simulink model "Alternative_VTOLAutopilotController"  (R2026a)
settings: configuration reference "VTOLConfiguration" (kept outside this file)
undefined symbols (not defined in the file): control, controlParams, ControlSampleTime, CriticalTiltAngle, DiscIntNeverNeededParam, dspblkCoreblockFVToolHelper, flightState, FSState, FWControlParams, FWTrimSpeed, gcbh, R_LOOKAHEAD, ReferenceFilterDen, ReferenceFilterNum, tilt_max, tilt_trim, tiltIni, TiltScheduleRate, uavParam, Vt, w_trim, WindDownRate, zGround
libraries: slpidlib x31, simulink x10, uavalgslib x7, simulink_extras x1, sl_discontinuities x1
(part 6 of 6)

== system Alternative_VTOLAutopilotController/Low level controller/Fixed Wing Controller/Fixed Wing Controller Module/Fixed Wing Controller Tuning/Attitude Controller/Pitch Roll Controller/Turn Coordinator ==
  Roll SP : Inport
  Pitch SP : Inport  Port=2
  Airspeed : Inport  Port=3
  r : Inport  Port=4
  MATLAB Function : MATLAB Function  TreatAsAtomicUnit=on
  Rudder Controller : slpidlib/PID Controller  Controller=P  Form=Parallel  TimeDomain=Discrete-time  UseExternalTs=off  SampleTime=-1  IntegratorMethod=Forward Euler  FilterMethod=Forward Euler  ControllerParametersSource=internal  P=0.01  I=1  UseKiTs=off  D=0  UseExternalDerivativeSource=off  N=100  UseFilter=on  TunerSelectOption=Transfer Function Based (PID Tuner App)  InitialConditionSource=internal  InitialConditionForIntegrator=0  InitialConditionForFilter=0  DifferentiatorICPrevScaledInput=0  ExternalReset=none  TrackingMode=off  Kt=1  LimitOutput=on  SatLimitsSource=internal  UpperSaturationLimit=1  LowerSaturationLimit=-1  LinearizeAsGain=on  AntiWindupMode=none  Kb=1  LimitIntegrator=off  UpperIntegratorSaturationLimit=inf  LowerIntegratorSaturationLimit=-inf  POutMin=[]  POutMax=[]  IOutMin=[]  IOutMax=[]  DOutMin=[]  DOutMax=[]  NOutMin=[]  NOutMax=[]  SumOutMin=[]  SumOutMax=[]  SaturationOutMin=[]  SaturationOutMax=[]  PParamMin=[]  PParamMax=[]  IParamMin=[]  IParamMax=[]  DParamMin=[]  DParamMax=[]  NParamMin=[]  NParamMax=[]  KbParamMin=[]  KbParamMax=[]  KtParamMin=[]  KtParamMax=[]  KbOutMin=[]  KbOutMax=[]  KtOutMin=[]  KtOutMax=[]  IntegratorOutMin=[]  IntegratorOutMax=[]  FilterOutMin=[]  FilterOutMax=[]  SumI1OutMin=[]  SumI1OutMax=[]  SumI2OutMin=[]  SumI2OutMax=[]  SumI3OutMin=[]  SumI3OutMax=[]  SumI4OutMin=[]  SumI4OutMax=[]  SumDOutMin=[]  SumDOutMax=[]  DifferentiatorOutMin=[]  DifferentiatorOutMax=[]  FilterDiffOutCoefMin=[]  FilterDiffOutCoefMax=[]  ReciprocalOutMin=[]  ReciprocalOutMax=[]  SumDenOutMin=[]  SumDenOutMax=[]  SumNumOutMin=[]  SumNumOutMax=[]  DivideOutMin=[]  DivideOutMax=[]  UdiffTsProdOutMin=[]  UdiffTsProdOutMax=[]  NTsProdOutMin=[]  NTsProdOutMax=[]  UintegralTsProdOutMin=[]  UintegralTsProdOutMax=[]  UngainTsProdOutMin=[]  UngainTsProdOutMax=[]  ClampingZeroOutDataTypeStr=Inherit: Inherit via back propagation  ClampingZeroOutMin=[]  ClampingZeroOutMax=[]  FilterDenConstantOutDataTypeStr=Inherit: Inherit via back propagation  FilterDenConstantOutMin=[]  FilterDenConstantOutMax=[]  PCopyOutDataTypeStr=Inherit: Inherit via back propagation  PCopyOutMin=[]  PCopyOutMax=[]  NCopyOutDataTypeStr=Inherit: Inherit via back propagation  NCopyOutMin=[]  NCopyOutMax=[]  IntegratorContinuousStateAttributes=''  IntegratorStateMustResolveToSignalObject=off  IntegratorRTWStateStorageClass=Auto  FilterContinuousStateAttributes=''  FilterStateMustResolveToSignalObject=off  FilterRTWStateStorageClass=Auto  ParallelPVariant=InternalParameters  IdealPVariant=Disabled  IVariant=Disabled  DVariant=Disabled  IntegratorVariant=Disabled  SatVariant=Enabled  AWVariant=Disabled  PCopyVariant=Disabled  TRVariant=Disabled  FdbkBlocksVariant=Forward  IdealPFdbkVariant=Disabled  SatFdbkVariant=Disabled  DerivativeFilterVariant=Disabled  NVariant=Disabled  NCopyVariant=Disabled_SignalSpec  FilterICVariant=Disabled  IntegratorICVariant=Disabled  ExternalResetVariant=Disabled  TRSumVariant=Passthrough  SumFdbkVariant=Disabled  SumVariant=Passthrough_P  TsampFilterVariant=InternalTs  TsampNgainVariant=Passthrough  TsampIntegralVariant=Disabled_SignalSpec  ExternalSaturationOutDataTypeStr=Inherit: Same as second input  DerivativeSourceVariant=Disabled  PreIntVariant=InternalPreInt
  Sum : Sum  Inputs=|+-
  Rudder : Outport
  wires:
  Roll SP/1 -> MATLAB Function/1(rollSP)
  Pitch SP/1 -> MATLAB Function/2(pitchSP)
  Airspeed/1 -> MATLAB Function/3(airSpeed)
  Sum/1 -> Rudder Controller/1
  Rudder Controller/1 -> Rudder/1
  r/1 -> Sum/2  "r"
  MATLAB Function/1(rSP) -> Sum/1  "rSP"

== system Alternative_VTOLAutopilotController/Guidance Test Bench/ControlType/Guidance Testbench/Guidance Logic/Guidance Stateflow/Guidance Mode Selector/GuidanceLogic.WP/Back Transition Guard/Triggered Subsystem ==
  Poses : Inport
  Trigger : TriggerPort  VariantControl=(inherit)
  Reshape : Reshape  OutputDimensionality=Customize  OutputDimensions=[3,1]
  Selector : Selector  InputPortWidth=4  IndexOptions=Index vector (dialog)  Indices=[1 2 3]  OutputSizes=1
  HoldPositionValue : Outport
  wires:
  Poses/1 -> Selector/1
  Selector/1 -> Reshape/1
  Reshape/1 -> HoldPositionValue/1

== system Alternative_VTOLAutopilotController/Guidance Test Bench/ControlType/Guidance Testbench/Guidance Logic/Guidance Stateflow/Guidance Mode Selector/GuidanceLogic.WP/Dist2WP/Subsystem ==
  V : Inport
  Dot Product1 : DotProduct  OutDataTypeStr=Inherit: Inherit via internal rule
  Product : Product  Inputs=*/
  Saturation : Saturate  UpperLimit=inf  LowerLimit=0.00001
  Sqrt : Sqrt
  V_unit : Outport
  wires:
  V/1 -> Dot Product1/2, Dot Product1/1, Product/1
  Sqrt/1 -> Product/2
  Dot Product1/1 -> Saturation/1
  Saturation/1 -> Sqrt/1
  Product/1 -> V_unit/1

== matlab function Alternative_VTOLAutopilotController/Guidance Test Bench/ControlType/Guidance Testbench/Guidance Logic/Guidance Stateflow/Guidance Mode Selector/GuidanceLogic.Land.ToLand/MATLAB Function ==
  data: FromWP input Bus: doubleUavPathManager size=1; wps output; ToWP input Bus: doubleUavPathManager size=1
function wps = getLandingWaypoint(FromWP, ToWP)

persistent outWPS

if isempty(outWPS)
    outWPS = double(zeros(2,4));
end

outWPS(1,:) = [FromWP.position' FromWP.params(4)];
outWPS(2,:) = [ToWP.position(1:2)' FromWP.position(3) ToWP.params(4)];

wps = outWPS;

== matlab function Alternative_VTOLAutopilotController/Guidance Test Bench/ControlType/Guidance Testbench/Guidance Logic/Guidance Stateflow/Guidance Mode Selector/GuidanceLogic.Land.Descend/MATLAB Function ==
  data: FromWP input Bus: doubleUavPathManager size=1; wps output; ToWPPos input size=[3 1]; ToWPParam input size=[4 1]
function wps = getLandingWaypoint(FromWP, ToWPPos, ToWPParam)

persistent outWPS

if isempty(outWPS)
    outWPS = double(zeros(2,4));
end

outWPS(1,:) = [FromWP.position' FromWP.params(4)];
outWPS(2,:) = [reshape(ToWPPos,1,[]), ToWPParam(4)];

wps = outWPS;

== matlab function Alternative_VTOLAutopilotController/Low level controller/Fixed Wing Controller/Fixed Wing Controller Module/Fixed Wing Controller Simulation/Attitude Controller/Pitch Roll Controller/Turn Coordinator/MATLAB Function ==
  data: rollSP input; rSP output; pitchSP input; airSpeed input
function rSP = fcn(rollSP, pitchSP, airSpeed)
    yawRateSP = tan(rollSP)*9.81/max(airSpeed,5);
    rSP = yawRateSP*cos(pitchSP)*cos(rollSP);
end

== matlab function Alternative_VTOLAutopilotController/Low level controller/Fixed Wing Controller/Fixed Wing Controller Module/Fixed Wing Controller Simulation/Lateral Guidance Logic/MATLAB Function ==
  data: courseSP input; lacc output; course input; rollSP output; groundSpeed input; L1 input
function [lacc, rollSP] = fcn(courseSP, course, groundSpeed, L1)
eta = courseSP - course;

% wrap -pi to pi
eta = mod(eta, 2*pi);
if eta>pi
    eta = eta - 2*pi;
end

% cap eta to -pi/2 to pi/2
eta = min(eta, pi/2);
eta = max(eta, -pi/2);

lacc = 2*(groundSpeed^2)/L1*sin(eta);

rollSP = atan(lacc/9.81);

== matlab function Alternative_VTOLAutopilotController/Low level controller/Fixed Wing Controller/Fixed Wing Controller Module/Fixed Wing Controller Tuning/Subsystem2/MATLAB Function ==
  data: phi input; y output; theta input
function y = fcn(phi,theta)

y=zeros(3,3);
y=[1 sin(phi)*tan(theta) cos(phi)*tan(theta); 0 cos(phi) -sin(phi); 0 sin(phi)/cos(theta) cos(phi)/cos(theta)];
end

== matlab function Alternative_VTOLAutopilotController/Low level controller/Fixed Wing Controller/Fixed Wing Controller Module/Fixed Wing Controller Tuning/Lateral Guidance Logic/MATLAB Function ==
  data: courseSP input; lacc output; course input; rollSP output; groundSpeed input; L1 input
function [lacc, rollSP] = fcn(courseSP, course, groundSpeed, L1)
eta = courseSP - course;

% wrap -pi to pi
eta = mod(eta, 2*pi);
if eta>pi
    eta = eta - 2*pi;
end

% cap eta to -pi/2 to pi/2
eta = min(eta, pi/2);
eta = max(eta, -pi/2);

lacc = 2*(groundSpeed^2)/L1*sin(eta);

rollSP = atan(lacc/9.81);

== matlab function Alternative_VTOLAutopilotController/Low level controller/Fixed Wing Controller/Fixed Wing Controller Module/Fixed Wing Controller Tuning/Attitude Controller/Pitch Roll Controller/Turn Coordinator/MATLAB Function ==
  data: rollSP input; rSP output; pitchSP input; airSpeed input
function rSP = fcn(rollSP, pitchSP, airSpeed)
    yawRateSP = tan(rollSP)*9.81/max(airSpeed,5);
    rSP = yawRateSP*cos(pitchSP)*cos(rollSP);
end

== matlab function Alternative_VTOLAutopilotController/Guidance Test Bench/ControlType/Guidance Testbench/Guidance Logic/Guidance Stateflow/Guidance Mode Selector/GuidanceLogic.BackTransition.BackTransition/MATLAB Function ==
  data: Vb input; tilt input; flag output
function flag = fcn(Vb,tilt)
tiltConditionMet=abs(tilt)<1e-1;
velocityConditionMet=abs(norm([Vb(1) 0 0]))<4;

flag=tiltConditionMet&velocityConditionMet;
end

== stateflow chart Alternative_VTOLAutopilotController/Guidance Test Bench/ControlType/Guidance Testbench/Guidance Logic/Guidance Stateflow/Guidance Mode Selector ==
  settings: updateMethod=DISCRETE  sampleTime=UAVSampleTime*4
  state GuidanceLogic
    state FIXED_WING_WAYPOINT
      en:
      controlMode.airspeedAltitude = 1;
      controlMode.attitude = 1;
      controlMode.lateralGuidance = 1;
      state WAYPOINT
    state FIXED_WING_ENTRY
      state Stabilize
        en:
        FlightMode=flightState.FixedWing;
        controlMode.attitude = 1;
        controlMode.airspeedAltitude = 0;
        controlMode.lateralGuidance = 0;
        %Transition once done.
        FixedWingSP.yaw = 0;
        FixedWingSP.pitch = 0;
        FixedWingSP.roll = 0;
        FixedWingSP.airspeed=14;
        Status= uint8(0);
      state FIXEDWINGFLIGHT
        en:
        % Control mode
        controlMode.airspeedAltitude = 1;
        controlMode.attitude = 1;
        controlMode.lateralGuidance = 1;
        % Setpoint init
        aacSP.L1 = 25;
        aacSP.airspeed = 14;
        aacSP.altitude = 0;
        aacSP.course=0;
      (default) -> Stabilize
      Stabilize -> FIXEDWINGFLIGHT : after(3,sec)
    state Start
      en:
      %Set Flight mode to hover
      FlightMode=PresetMode;
      %Set default settings
      % Control mode
      controlMode.airspeedAltitude = 0;
      controlMode.attitude = 0;
      controlMode.lateralGuidance = 0;
      controlMode.TransitionCondition = 0;
      % Setpoint init
      FixedWingSP.yaw = 0;
      FixedWingSP.pitch = 0;
      FixedWingSP.roll = 0;
      FixedWingSP.airspeed=14;
      aacSP.L1 = 25;
      aacSP.airspeed = 14;
      aacSP.altitude = 0;
      aacSP.course=0;
      InnerLoopCmds.YawCmd=0;
    state FIXED_WING_ORBIT
      en:
      controlMode.airspeedAltitude = 1;
      controlMode.attitude = 1;
      controlMode.lateralGuidance = 1;
      state ORBIT
    state HOVER_ENTRY
      en:
      FlightMode=flightState.Hover;
      controlMode.inTransition=0;
    state Takeoff
    state WP
    state Orbit
    state PreTransition
      en:
      FlightMode=flightState.FixedWing;
      controlMode.airspeedAltitude = 1;
      controlMode.attitude = 1;
      controlMode.lateralGuidance = 1;
      % Setpoint init
      aacSP.L1 = 25;
      aacSP.airspeed = 14;
      aacSP.altitude = altitudeHold;
      aacSP.course=courseHold;
    state BackTransition
      state BackTransition
    state ForwardTransition
    state FWCOMPLETE
      Status=uint8(1);
      controlMode.TransitionCondition=uint8(1);
    note: [(mode==4)]
    state Land
      state Descend
      state ToLand
      (default) -> ToLand
      ToLand -> Descend : [(norm(Pose(1:2)-ToWP.position(1:2)) <= 3)]
    (default) -> Start
    Start -> (junction 5)
    FIXEDWINGFLIGHT -> WAYPOINT [order 2] : [(mode==2)]
        | {Status=uint8(0);}
    FIXEDWINGFLIGHT -> ORBIT [order 1] : [(mode==3)]
        | {Status= uint8(0);}
    (junction 262) -> FIXED_WING_ENTRY
    (junction 5) -> FIXED_WING_ORBIT [order 6] : [(mode==3)&&(FlightMode==flightState.FixedWing)]
        | {Status=uint8(0);}
    (junction 5) -> (junction 262) [order 3] : [(FlightMode==flightState.Transition)]
        | {controlMode.inTransition=0;}
    (junction 255) -> HOVER_ENTRY
    (junction 5) -> (junction 255) [order 4] : [(FlightMode==flightState.BackTransition)]
        | {controlMode.inTransition=0;}
    HOVER_ENTRY -> (junction 12)
    (junction 257) -> FIXED_WING_WAYPOINT
    Takeoff -> WP : [Pose(3) <= ToWP.position(3)]{Status = uint8(1);}
    GuidanceLogic -> (junction 5) : [(hasChanged(mode))]
    (junction 5) -> Takeoff [order 5] : [(mode == 1)&&(FlightMode==flightState.Hover)]
        | {controlMode.inTransition=0;}
    (junction 5) -> (junction 257) [order 2] : [(mode==2)&&(FlightMode==flightState.FixedWing)]
        | {Status=uint8(0);}
    (junction 5) -> (junction 260) [order 1] : [(mode==6)&&(FlightMode==flightState.FixedWing)]
        | {courseHold=States.course;
        | altitudeHold=-States.Xe(3); }
    (junction 5) -> (junction 12) [order 7] : [FlightMode==flightState.Hover]
        | {controlMode.inTransition=0;}
    (junction 260) -> PreTransition
    (junction 12) -> WP [order 1] : [(mode==2)]
    (junction 12) -> (junction 17) [order 2]
    (junction 17) -> Orbit [order 1] : [(mode==3)]
    (junction 17) -> (junction 22) [order 2]
    PreTransition -> GuidanceLogic.BackTransition : after(5,sec)
        | {FlightMode=flightState.BackTransition;
        | controlMode.inTransition=1; }
    (junction 22) -> ForwardTransition [order 1] : [(mode==6)]
        | {FlightMode=flightState.Transition;
        | controlMode.inTransition=1;
        | controlMode.TransitionCondition=uint8(0);
        |
        | }
    (junction 22) -> Land [order 2]
    ForwardTransition -> FWCOMPLETE : [transitionConditionMet(States,Vt)]
  (default) -> GuidanceLogic
  data: sf_internal_action_state_placeholder_data local double size=1 =0; sf_internal_action_state_placeholder_data local double size=1 =0; sf_internal_action_state_placeholder_data local double size=1 =0; sf_internal_action_state_placeholder_data local double size=1 =0; sf_internal_action_state_placeholder_data local double size=1 =0; sf_internal_action_state_placeholder_data local double size=1 =0; sf_internal_action_state_placeholder_data local double size=1 =0; sf_internal_action_state_placeholder_data local double size=1 =0; sf_internal_action_state_placeholder_data local double size=1 =0; TransitionSt function_input Bus: GuidanceStates; valid function_output; Vtransition function_input; mode input; ToWP input Bus: doubleUavPathManager; Status output uint8; FromWP input Bus: doubleUavPathManager; Pose input; GdncMode output Enum: GdncModeType; States input; aacSP output Bus: AAC; FixedWingSP output Bus: FixedWingCommandBus; controlMode output Bus: controlMode; FlightMode output; PresetMode input; courseHold local; altitudeHold local; Vt parameter double; InnerLoopCmds output Bus: innerLoopCmdsBus; zGround parameter; Ground input
  function valid=transitionConditionMet(TransitionSt,Vtransition):
    | function valid=transitionConditionMet(TransitionSt,Vtransition)
    | %wingsLevel
    | if(States.Tilt>=1.57)&&(vecnorm(States.Ve)>Vt)
    |    valid=true;
    | else
    |     valid=false;
    | end
    | end

== matlab function Alternative_VTOLAutopilotController/Guidance Test Bench/ControlType/Guidance Testbench/Guidance Logic/Guidance Stateflow/Guidance Mode Selector/GuidanceLogic.WP/MATLAB Function ==
  data: FromWP input Bus: doubleUavPathManager size=1; wps output; ToWP input Bus: doubleUavPathManager size=1
function wps = getWaypointMission(FromWP, ToWP)

persistent outWPS

if isempty(outWPS)
    outWPS = double(zeros(2,4));
end

outWPS(1,:) = [FromWP.position' FromWP.params(4)];
outWPS(2,:) = [ToWP.position' ToWP.params(4)];

wps = outWPS;

== matlab function Alternative_VTOLAutopilotController/Guidance Test Bench/ControlType/Guidance Testbench/Guidance Logic/Guidance Stateflow/Guidance Mode Selector/GuidanceLogic.FIXED_WING_WAYPOINT.WAYPOINT/MATLAB Function ==
  data: toWP input; wps output; fromWP input; alt output
function [wps, alt]= fcn(toWP, fromWP)
    wps = zeros(2,3); %#ok<PREALL> 
    wps = [fromWP'; toWP'];
    alt = -toWP(3);
end

== matlab function Alternative_VTOLAutopilotController/Low level controller/Fixed Wing Controller/Fixed Wing Controller Module/Fixed Wing Controller Simulation/Subsystem2/MATLAB Function ==
  data: phi input; y output; theta input
function y = fcn(phi,theta)

y=zeros(3,3);
y=[1 sin(phi)*tan(theta) cos(phi)*tan(theta); 0 cos(phi) -sin(phi); 0 sin(phi)/cos(theta) cos(phi)/cos(theta)];
end

== stateflow chart Alternative_VTOLAutopilotController/Guidance Test Bench/ControlType/Manual Control/Command Interface/Basic Control  Switching ==
  state STATE_MACHINE
    state DEFAULT
      en:
      controlMode.lateralGuidance=1;
      controlMode.airspeedAltitude=1;
      controlMode.attitude=1;
      controlMode.manual=0;
      controlMode.armed=0;
      controlMode.inTransition=0;
    state TRANSITION
      controlMode.lateralGuidance=1;
      controlMode.airspeedAltitude=1;
      controlMode.attitude=1;
      controlMode.manual=0;
      controlMode.armed=0;
      controlMode.inTransition=1;
      controlMode.TransitionCondition=0;
    (default) -> DEFAULT
    STATE_MACHINE -> DEFAULT [order 2] : [hasChanged(FlightMode)]
    STATE_MACHINE -> TRANSITION [order 1] : [hasChanged(FlightMode)&&((FlightMode==flightState.Transition)||(FlightMode==flightState.BackTransition))]
    TRANSITION -> STATE_MACHINE [order 2] : [backConditioMet(States)&&(FlightMode==flightState.BackTransition)]
        | {controlMode.TransitionCondition=1;
        | controlMode.inTransition=0;}
    TRANSITION -> STATE_MACHINE [order 1] : [transitionConditionMet(States,Vt)&&(FlightMode==flightState.Transition)]
        | {controlMode.TransitionCondition=1;
        | controlMode.inTransition=0;}
  data: TransitionStates function_input Bus: GuidanceStates; valid function_output; Vtransition function_input; TransitionStates function_input Bus: GuidanceStates; valid function_output; controlMode output Bus: controlMode; FlightMode input; States input; Vt parameter double
  function valid=transitionConditionMet(TransitionStates,Vtransition):
    | function valid=transitionConditionMet(TransitionStates,Vtransition)
    | %wingsLevel
    | if((States.Tilt>=1.57)&&(vecnorm(States.Ve)>Vt))
    |    valid=true;
    | else
    |     valid=false;
    | end
    | end
  function valid=backConditioMet(TransitionStates):
    | function valid=backConditioMet(TransitionStates)
    | %wingsLevel
    | if(vecnorm(States.Ve)<1e-1)
    |    valid=true;
    | else
    |     valid=false;
    | end
    | end
